simulink model "project1_sim"  (R2022b)
settings: Solver=VariableStepAuto  StartTime=0.0  StopTime=10.0  RelTol=1e-3
settings Model: Creator=hayden  LastModifiedBy=hayden

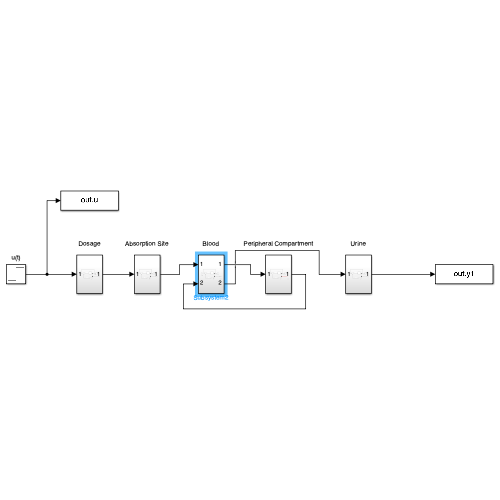
[thumbnail: Simulink's stored preview of the top-level diagram]
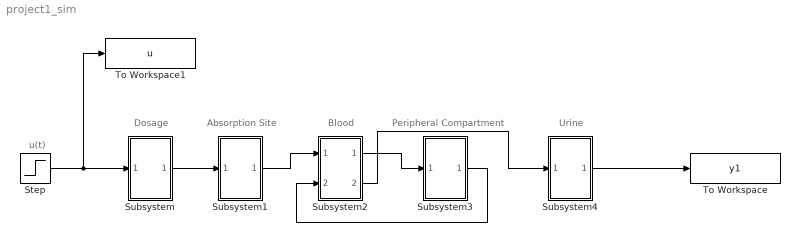
== system project1_sim ==
  note: Urine
  note: Peripheral Compartment
  note: Blood
  note: Absorption Site
  note: Dosage
  note: u(t)
  Step : Step  Time=0  SampleTime=0
  Subsystem : Subsystem
  Subsystem1 : Subsystem
  Subsystem2 : Subsystem
  Subsystem3 : Subsystem
  Subsystem4 : Subsystem
  To Workspace : ToWorkspace  VariableName=y1  SaveFormat=Timeseries  SampleTime=-1
  To Workspace1 : ToWorkspace  VariableName=u  SaveFormat=Timeseries  SampleTime=-1
  wires:
  Step/1 -> To Workspace1/1, Subsystem/1(In1)
  Subsystem/1(Out1) -> Subsystem1/1(In1)
  Subsystem1/1(Out1) -> Subsystem2/1(In1)
  Subsystem2/1(Out1) -> Subsystem3/1(In1)
  Subsystem3/1(Out2) -> Subsystem2/2(In2)
  Subsystem2/2(Out2) -> Subsystem4/1(In1)
  Subsystem4/1(Out1) -> To Workspace/1

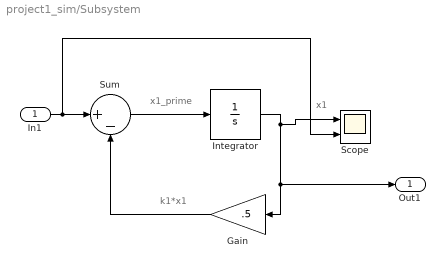
== system project1_sim/Subsystem ==
  note: k1*x1
  note: x1
  note: x1_prime
  In1 : Inport
  Gain : Gain  Gain=.5
  Integrator : Integrator
  Scope : Scope  NumInputPorts=2
  Sum : Sum  Inputs=|+-
  Out1 : Outport
  wires:
  In1/1 -> Scope/2, Sum/1
  Gain/1 -> Sum/2
  Sum/1 -> Integrator/1
  Integrator/1 -> Out1/1, Gain/1, Scope/1

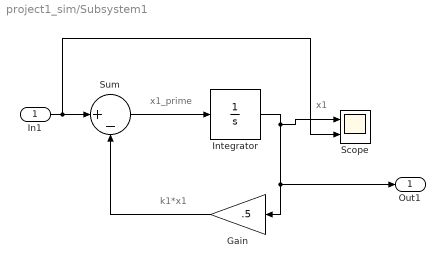
== system project1_sim/Subsystem1 ==
  note: k1*x1
  note: x1
  note: x1_prime
  In1 : Inport
  Gain : Gain  Gain=.5
  Integrator : Integrator
  Scope : Scope  NumInputPorts=2
  Sum : Sum  Inputs=|+-
  Out1 : Outport
  wires:
  In1/1 -> Scope/2, Sum/1
  Gain/1 -> Sum/2
  Sum/1 -> Integrator/1
  Integrator/1 -> Out1/1, Gain/1, Scope/1

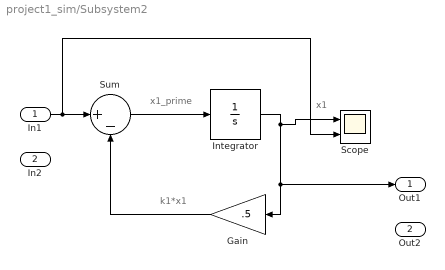
== system project1_sim/Subsystem2 ==
  note: k1*x1
  note: x1
  note: x1_prime
  In1 : Inport
  In2 : Inport  Port=2
  Gain : Gain  Gain=.5
  Integrator : Integrator
  Scope : Scope  NumInputPorts=2
  Sum : Sum  Inputs=|+-
  Out1 : Outport
  Out2 : Outport  Port=2
  wires:
  In1/1 -> Scope/2, Sum/1
  Gain/1 -> Sum/2
  Sum/1 -> Integrator/1
  Integrator/1 -> Out1/1, Gain/1, Scope/1

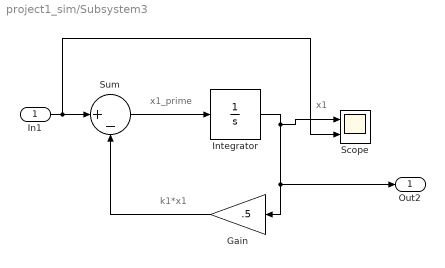
== system project1_sim/Subsystem3 ==
  note: k1*x1
  note: x1
  note: x1_prime
  In1 : Inport
  Gain : Gain  Gain=.5
  Integrator : Integrator
  Scope : Scope  NumInputPorts=2
  Sum : Sum  Inputs=|+-
  Out2 : Outport
  wires:
  In1/1 -> Scope/2, Sum/1
  Gain/1 -> Sum/2
  Sum/1 -> Integrator/1
  Integrator/1 -> Out2/1, Gain/1, Scope/1

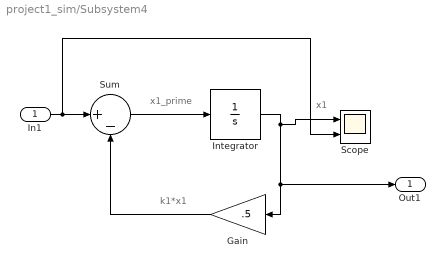
== system project1_sim/Subsystem4 ==
  note: k1*x1
  note: x1
  note: x1_prime
  In1 : Inport
  Gain : Gain  Gain=.5
  Integrator : Integrator
  Scope : Scope  NumInputPorts=2
  Sum : Sum  Inputs=|+-
  Out1 : Outport
  wires:
  In1/1 -> Scope/2, Sum/1
  Gain/1 -> Sum/2
  Sum/1 -> Integrator/1
  Integrator/1 -> Out1/1, Gain/1, Scope/1
